simulink model "modelo_protyecot"  (R2024b)
settings: Solver=VariableStepAuto  StartTime=0.0  StopTime=10.0  RelTol=1e-3
undefined symbols (not defined in the file): b_p, g, J, k, L_barra, L_cm_helice, m_barra, m_helice_motor, x1_0, x2_0
settings Model: Creator=juanm  LastModifiedBy=juanm

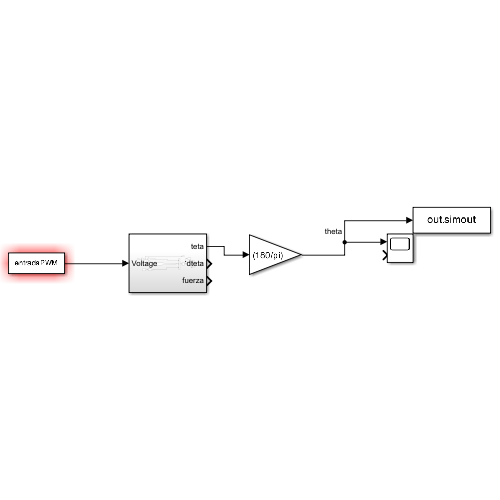
[thumbnail: Simulink's stored preview of the top-level diagram]
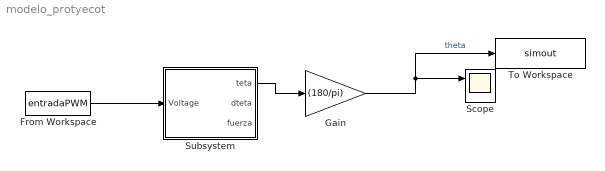
== system modelo_protyecot ==
  From Workspace : FromWorkspace  VariableName=entradaPWM
  Gain : Gain  Gain=(180/pi)
  Scope : Scope  NumInputPorts=2
  Subsystem : Subsystem
  To Workspace : ToWorkspace  VariableName=simout  SaveFormat=Timeseries  SampleTime=-1
  wires:
  Gain/1 -> To Workspace/1, Scope/1  "theta"
  Subsystem/1(teta) -> Gain/1
  From Workspace/1 -> Subsystem/1(Voltage)

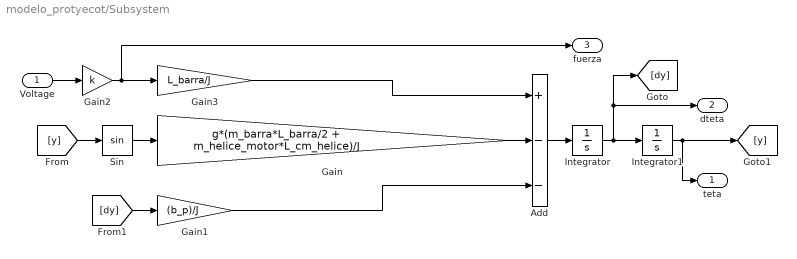
== system modelo_protyecot/Subsystem ==
  Voltage : Inport
  Add : Sum  Inputs=+--
  Gain : Gain  Gain=g*(m_barra*L_barra/2 + m_helice_motor*L_cm_helice)/J
  Gain1 : Gain  Gain=(b_p)/J
  Gain2 : Gain  Gain=k
  Gain3 : Gain  Gain=L_barra/J
  Integrator : Integrator  InitialCondition=x2_0
  Integrator1 : Integrator  InitialCondition=x1_0
  Sin : Trigonometry
  teta : Outport
  dteta : Outport  Port=2
  fuerza : Outport  Port=3
  wires:
  Integrator/1 -> [dy], dteta/1, Integrator1/1
  [dy] -> Gain1/1
  Add/1 -> Integrator/1
  Sin/1 -> Gain/1
  Gain/1 -> Add/2
  [y] -> Sin/1
  Gain1/1 -> Add/3
  Voltage/1 -> Gain2/1
  Gain2/1 -> fuerza/1, Gain3/1
  Gain3/1 -> Add/1
  Integrator1/1 -> [y], teta/1
